simulink library "LIB_Quad_Com"  (Simulink 7.6)
settings: Solver=ode45  StartTime=0.0  StopTime=10.0  RelTol=1e-3
libraries: simulink x5
settings Model: Creator=Thomas  LastModifiedBy=Administrator

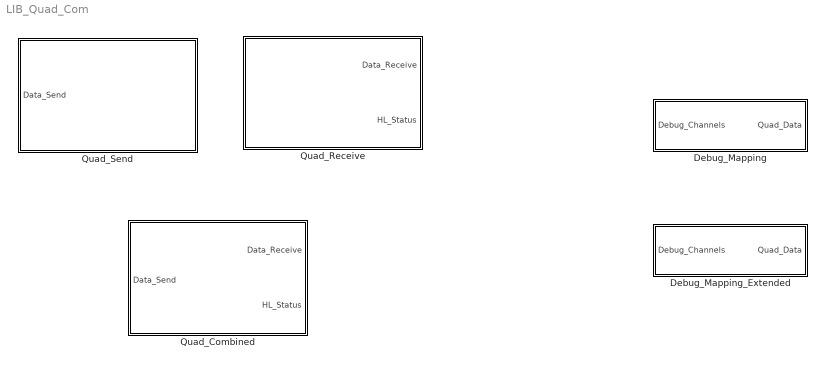
== system LIB_Quad_Com ==
  Debug_Mapping : Subsystem
  Debug_Mapping_Extended : Subsystem
  Quad_Combined : Subsystem  mask{baudrate=250000}
      mask Display:
      | image(imread('hummingbird.jpg'),[.15, .15, .7, .7],'on'),
      | port_label('input',1,'u'),
      | port_label('output',1,'y'),
      | port_label('output',2,'Status')
  Quad_Receive : Subsystem  mask{baudrate=250000}
      mask Display:
      | image(imread('hummingbird.jpg'),[.15, .15, .7, .7],'on'),
      | port_label('output',1,'y'),
      | port_label('output',2,'Status')
  Quad_Send : Subsystem  mask{baudrate=250000}
      mask Display:
      | image(imread('hummingbird.jpg'),[.15, .15, .7, .7],'on'),
      | port_label('input',1,'u')

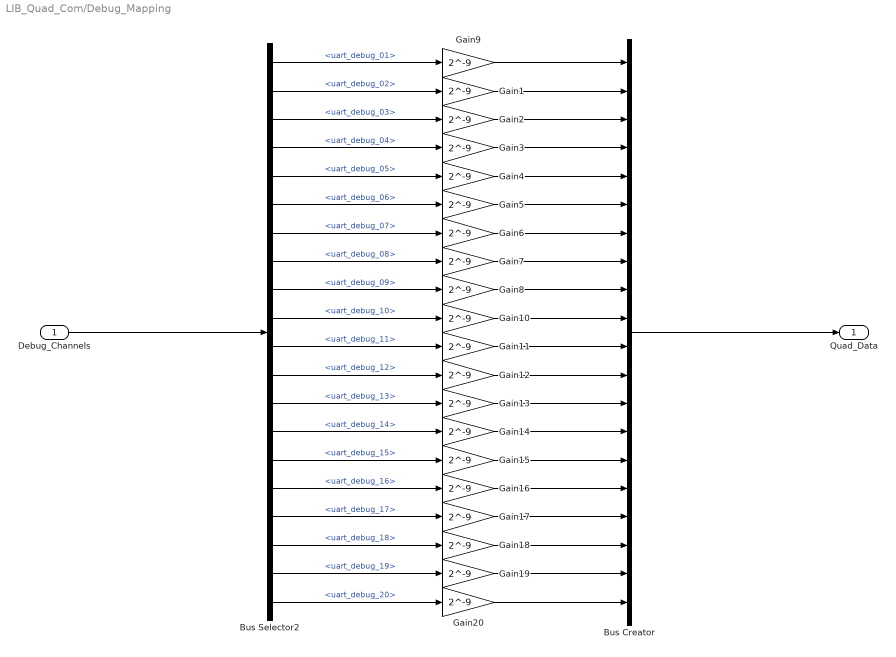
== system LIB_Quad_Com/Debug_Mapping ==
  Debug_Channels : Inport
  Bus Creator : BusCreator  Inputs=20
  Bus Selector2 : BusSelector  OutputSignals=uart_debug_01,uart_debug_02,uart_debug_03,uart_debug_04,uart_debug_05,uart_debug_06,uart_debug_07,uart_debug_08,uart_debug_09,uart_debug_10,uart_debug_11,uart_debug_12,uart_debug_13,uart_debug_14,uart_debug_15,uart_debug_16,uart_debug_17,uart_debug_18,uart_debug_19,uart_debug_20
  Gain{1..20} (20 alike) : Gain  Gain=2^-9  OutDataTypeStr=double
  Quad_Data : Outport
  wires:
  Gain20/1 -> Bus Creator/20
  Gain19/1 -> Bus Creator/19
  Gain18/1 -> Bus Creator/18
  Gain17/1 -> Bus Creator/17
  Gain16/1 -> Bus Creator/16
  Gain15/1 -> Bus Creator/15
  Gain14/1 -> Bus Creator/14
  Gain13/1 -> Bus Creator/13
  Gain12/1 -> Bus Creator/12
  Gain11/1 -> Bus Creator/11
  Gain10/1 -> Bus Creator/10
  Gain8/1 -> Bus Creator/9
  Gain7/1 -> Bus Creator/8
  Gain6/1 -> Bus Creator/7
  Gain5/1 -> Bus Creator/6
  Gain4/1 -> Bus Creator/5
  Gain3/1 -> Bus Creator/4
  Gain2/1 -> Bus Creator/3
  Gain1/1 -> Bus Creator/2
  Gain9/1 -> Bus Creator/1
  Bus Selector2/20 -> Gain20/1  "<uart_debug_20>"
  Bus Selector2/19 -> Gain19/1  "<uart_debug_19>"
  Bus Selector2/18 -> Gain18/1  "<uart_debug_18>"
  Bus Selector2/17 -> Gain17/1  "<uart_debug_17>"
  Bus Selector2/16 -> Gain16/1  "<uart_debug_16>"
  Bus Selector2/15 -> Gain15/1  "<uart_debug_15>"
  Bus Selector2/14 -> Gain14/1  "<uart_debug_14>"
  Bus Selector2/13 -> Gain13/1  "<uart_debug_13>"
  Bus Selector2/12 -> Gain12/1  "<uart_debug_12>"
  Bus Selector2/11 -> Gain11/1  "<uart_debug_11>"
  Bus Selector2/10 -> Gain10/1  "<uart_debug_10>"
  Bus Selector2/9 -> Gain8/1  "<uart_debug_09>"
  Bus Selector2/8 -> Gain7/1  "<uart_debug_08>"
  Bus Selector2/7 -> Gain6/1  "<uart_debug_07>"
  Bus Selector2/6 -> Gain5/1  "<uart_debug_06>"
  Bus Selector2/5 -> Gain4/1  "<uart_debug_05>"
  Bus Selector2/4 -> Gain3/1  "<uart_debug_04>"
  Bus Selector2/3 -> Gain2/1  "<uart_debug_03>"
  Bus Selector2/2 -> Gain1/1  "<uart_debug_02>"
  Bus Selector2/1 -> Gain9/1  "<uart_debug_01>"
  Debug_Channels/1 -> Bus Selector2/1
  Bus Creator/1 -> Quad_Data/1

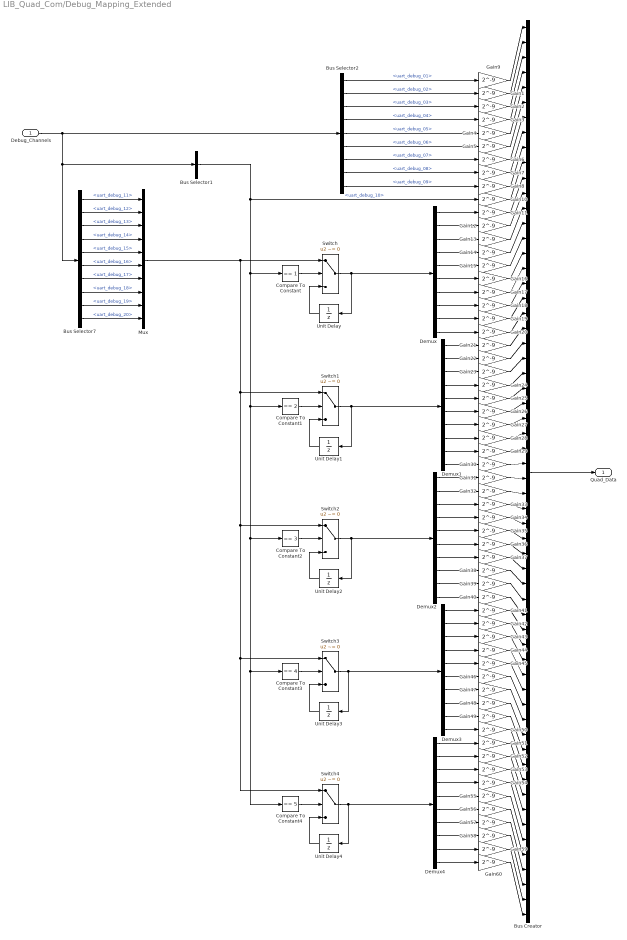
== system LIB_Quad_Com/Debug_Mapping_Extended ==
  Debug_Channels : Inport
  Bus Creator : BusCreator  Inputs=60
  Bus Selector1 : BusSelector  OutputSignals=uart_debug_10
  Bus Selector2 : BusSelector  OutputSignals=uart_debug_01,uart_debug_02,uart_debug_03,uart_debug_04,uart_debug_05,uart_debug_06,uart_debug_07,uart_debug_08,uart_debug_09
  Bus Selector7 : BusSelector  OutputSignals=uart_debug_11,uart_debug_12,uart_debug_13,uart_debug_14,uart_debug_15,uart_debug_16,uart_debug_17,uart_debug_18,uart_debug_19,uart_debug_20
  Compare To Constant : simulink/Logic and Bit Operations/Compare To Constant  SystemSampleTime=-1  relop===  const=1  LogicOutDataTypeMode=uint8  ZeroCross=off
  Compare To Constant1 : simulink/Logic and Bit Operations/Compare To Constant  SystemSampleTime=-1  relop===  const=2  LogicOutDataTypeMode=uint8  ZeroCross=off
  Compare To Constant2 : simulink/Logic and Bit Operations/Compare To Constant  SystemSampleTime=-1  relop===  const=3  LogicOutDataTypeMode=uint8  ZeroCross=off
  Compare To Constant3 : simulink/Logic and Bit Operations/Compare To Constant  SystemSampleTime=-1  relop===  const=4  LogicOutDataTypeMode=uint8  ZeroCross=off
  Compare To Constant4 : simulink/Logic and Bit Operations/Compare To Constant  SystemSampleTime=-1  relop===  const=5  LogicOutDataTypeMode=uint8  ZeroCross=off
  Demux{,1..4} (5 alike) : Demux  Outputs=10
  Gain{1..60} (60 alike) : Gain  Gain=2^-9  OutDataTypeStr=double
  Mux : Mux  Inputs=10
  Switch{,1..4} (5 alike) : Switch  Criteria=u2 ~= 0
  Unit Delay{,1..4} (5 alike) : UnitDelay  SampleTime=-1
  Quad_Data : Outport
  wires:
  Gain9/1 -> Bus Creator/1
  Bus Creator/1 -> Quad_Data/1
  Unit Delay4/1 -> Switch4/3
  Switch4/1 -> Demux4/1, Unit Delay4/1
  Compare To Constant4/1 -> Switch4/2
  Unit Delay3/1 -> Switch3/3
  Switch3/1 -> Demux3/1, Unit Delay3/1
  Compare To Constant3/1 -> Switch3/2
  Unit Delay2/1 -> Switch2/3
  Switch2/1 -> Demux2/1, Unit Delay2/1
  Compare To Constant2/1 -> Switch2/2
  Unit Delay1/1 -> Switch1/3
  Switch1/1 -> Demux1/1, Unit Delay1/1
  Compare To Constant1/1 -> Switch1/2
  Unit Delay/1 -> Switch/3
  Switch/1 -> Unit Delay/1, Demux/1
  Compare To Constant/1 -> Switch/2
  Demux4/10 -> Gain60/1
  Demux4/9 -> Gain59/1
  Demux4/8 -> Gain58/1
  Demux4/7 -> Gain57/1
  Demux4/6 -> Gain56/1
  Demux4/5 -> Gain55/1
  Demux4/4 -> Gain54/1
  Demux4/3 -> Gain53/1
  Demux4/2 -> Gain52/1
  Demux4/1 -> Gain51/1
  Demux3/10 -> Gain50/1
  Demux3/9 -> Gain49/1
  Demux3/8 -> Gain48/1
  Demux3/7 -> Gain47/1
  Demux3/6 -> Gain46/1
  Demux3/5 -> Gain45/1
  Demux3/4 -> Gain44/1
  Demux3/3 -> Gain43/1
  Demux3/2 -> Gain42/1
  Demux3/1 -> Gain41/1
  Demux2/10 -> Gain40/1
  Demux2/9 -> Gain39/1
  Demux2/8 -> Gain38/1
  Demux2/7 -> Gain37/1
  Demux2/6 -> Gain36/1
  Demux2/5 -> Gain35/1
  Demux2/4 -> Gain34/1
  Demux2/3 -> Gain33/1
  Demux2/2 -> Gain32/1
  Demux2/1 -> Gain31/1
  Demux1/10 -> Gain30/1
  Demux1/9 -> Gain29/1
  Demux1/8 -> Gain28/1
  Demux1/7 -> Gain27/1
  Demux1/6 -> Gain26/1
  Demux1/5 -> Gain25/1
  Demux1/4 -> Gain24/1
  Demux1/3 -> Gain23/1
  Demux1/2 -> Gain22/1
  Demux1/1 -> Gain21/1
  Demux/10 -> Gain20/1
  Demux/9 -> Gain19/1
  Demux/8 -> Gain18/1
  Demux/7 -> Gain17/1
  Demux/6 -> Gain16/1
  Demux/5 -> Gain15/1
  Demux/4 -> Gain14/1
  Demux/3 -> Gain13/1
  Demux/2 -> Gain12/1
  Demux/1 -> Gain11/1
  Bus Selector2/9 -> Gain8/1  "<uart_debug_09>"
  Bus Selector2/8 -> Gain7/1  "<uart_debug_08>"
  Bus Selector2/7 -> Gain6/1  "<uart_debug_07>"
  Bus Selector2/6 -> Gain5/1  "<uart_debug_06>"
  Bus Selector2/5 -> Gain4/1  "<uart_debug_05>"
  Bus Selector2/4 -> Gain3/1  "<uart_debug_04>"
  Bus Selector2/3 -> Gain2/1  "<uart_debug_03>"
  Bus Selector2/2 -> Gain1/1  "<uart_debug_02>"
  Bus Selector2/1 -> Gain9/1  "<uart_debug_01>"
  Bus Selector1/1 -> Compare To Constant4/1, Compare To Constant3/1, Compare To Constant2/1, Compare To Constant1/1, Compare To Constant/1, Gain10/1  "<uart_debug_10>"
  Mux/1 -> Switch4/1, Switch3/1, Switch2/1, Switch1/1, Switch/1
  Bus Selector7/10 -> Mux/10  "<uart_debug_20>"
  Bus Selector7/9 -> Mux/9  "<uart_debug_19>"
  Bus Selector7/8 -> Mux/8  "<uart_debug_18>"
  Bus Selector7/7 -> Mux/7  "<uart_debug_17>"
  Bus Selector7/6 -> Mux/6  "<uart_debug_16>"
  Bus Selector7/5 -> Mux/5  "<uart_debug_15>"
  Bus Selector7/4 -> Mux/4  "<uart_debug_14>"
  Bus Selector7/3 -> Mux/3  "<uart_debug_13>"
  Bus Selector7/2 -> Mux/2  "<uart_debug_12>"
  Bus Selector7/1 -> Mux/1  "<uart_debug_11>"
  Debug_Channels/1 -> Bus Selector1/1, Bus Selector7/1, Bus Selector2/1
  Gain1/1 -> Bus Creator/2
  Gain2/1 -> Bus Creator/3
  Gain3/1 -> Bus Creator/4
  Gain4/1 -> Bus Creator/5
  Gain5/1 -> Bus Creator/6
  Gain6/1 -> Bus Creator/7
  Gain7/1 -> Bus Creator/8
  Gain8/1 -> Bus Creator/9
  Gain10/1 -> Bus Creator/10
  Gain11/1 -> Bus Creator/11
  Gain12/1 -> Bus Creator/12
  Gain13/1 -> Bus Creator/13
  Gain14/1 -> Bus Creator/14
  Gain15/1 -> Bus Creator/15
  Gain16/1 -> Bus Creator/16
  Gain17/1 -> Bus Creator/17
  Gain18/1 -> Bus Creator/18
  Gain19/1 -> Bus Creator/19
  Gain20/1 -> Bus Creator/20
  Gain21/1 -> Bus Creator/21
  Gain22/1 -> Bus Creator/22
  Gain23/1 -> Bus Creator/23
  Gain24/1 -> Bus Creator/24
  Gain25/1 -> Bus Creator/25
  Gain26/1 -> Bus Creator/26
  Gain27/1 -> Bus Creator/27
  Gain28/1 -> Bus Creator/28
  Gain29/1 -> Bus Creator/29
  Gain30/1 -> Bus Creator/30
  Gain31/1 -> Bus Creator/31
  Gain32/1 -> Bus Creator/32
  Gain33/1 -> Bus Creator/33
  Gain34/1 -> Bus Creator/34
  Gain35/1 -> Bus Creator/35
  Gain36/1 -> Bus Creator/36
  Gain37/1 -> Bus Creator/37
  Gain38/1 -> Bus Creator/38
  Gain39/1 -> Bus Creator/39
  Gain40/1 -> Bus Creator/40
  Gain41/1 -> Bus Creator/41
  Gain42/1 -> Bus Creator/42
  Gain43/1 -> Bus Creator/43
  Gain44/1 -> Bus Creator/44
  Gain45/1 -> Bus Creator/45
  Gain46/1 -> Bus Creator/46
  Gain47/1 -> Bus Creator/47
  Gain48/1 -> Bus Creator/48
  Gain49/1 -> Bus Creator/49
  Gain50/1 -> Bus Creator/50
  Gain51/1 -> Bus Creator/51
  Gain52/1 -> Bus Creator/52
  Gain53/1 -> Bus Creator/53
  Gain54/1 -> Bus Creator/54
  Gain55/1 -> Bus Creator/55
  Gain56/1 -> Bus Creator/56
  Gain57/1 -> Bus Creator/57
  Gain58/1 -> Bus Creator/58
  Gain59/1 -> Bus Creator/59
  Gain60/1 -> Bus Creator/60

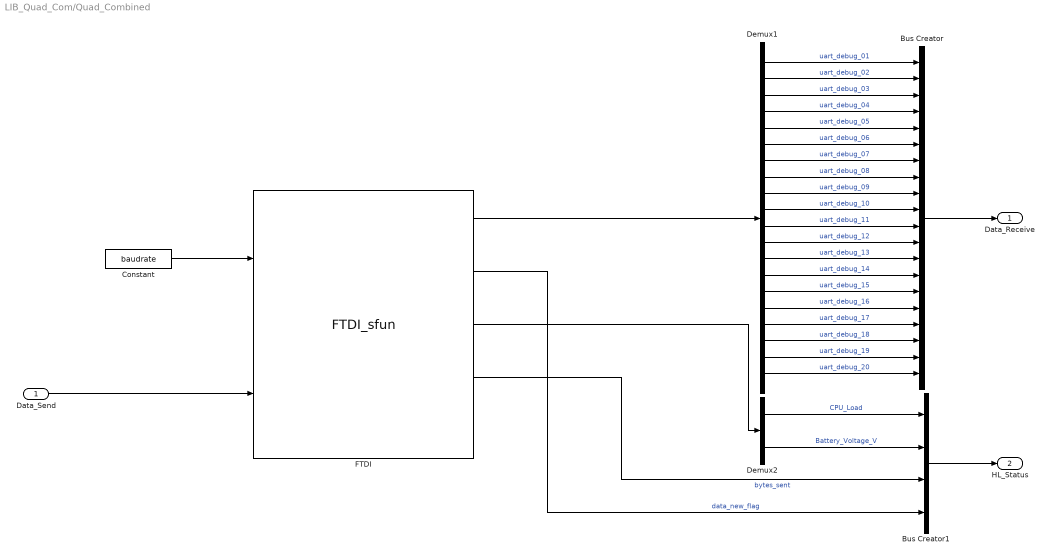
== system LIB_Quad_Com/Quad_Combined ==
  Data_Send : Inport  PortDimensions=[12 1]
  Bus Creator : BusCreator  Inputs=20
  Bus Creator1 : BusCreator
  Constant : Constant  Value=baudrate  OutDataTypeStr=int32  SampleTime=0.02
  Demux1 : Demux  Outputs=20
  Demux2 : Demux  Outputs=2
  FTDI : S-Function  InitFcn=try, set_param(gcb,'FunctionName','FTDI_sfun'), end  FunctionName=FTDI_sfun  SFunctionModules=FTDI_receive_sfun_wrapper ftditools  WizardData=DataTag0  EnableBusSupport=off  mask(S-Function Builder){}
      mask help: The S-Function Builder block creates a wrapper C-MEX S-function from your supplied C code with multiple input ports, output ports, and a variable number of scalar, vector, or matrix parameters. The input and output ports can propagate Simulink built-in data types, fixed-point datatypes, complex, frame, 1-D, and 2-D signals. This block also supports discrete and continuous states of type real. You can optionally have the block generate a TLC file to be used with Real-Time Workshop for code generation.
      mask init:
      | val = [[.9  0.75 0.75 1 1 .9 .9 1]',[1 1 0.75 0.75 .9 .9 1 .9]'];try , sys = get_param(gcb,'SfunBuilderFcnName');if isempty(sys), sys = get_param(gcb,'FunctionName'); end,catch, sys = get_param(gcb,'FunctionName'); end
      settings: CopyFcn=set_param(gcbh,'LinkStatus','none')  PreSaveFcn=try, set_param(gcb,'FunctionName','FTDI_sfun'), end  OpenFcn=sfunctionwizard(gcbh)
      mask Display: plot(val(:,1),val(:,2)),disp(sys), port_label('input',1,'set_BaudRate'), port_label('input',2,'data_send'), port_label('output',1,'data_out'), port_label('output',2,'data_new_flag'), port_label('output',3,'HL_Status'), port_label('output',4,'bytes_sent')
  Data_Receive : Outport
  HL_Status : Outport  Port=2
  wires:
  Data_Send/1 -> FTDI/2
  Constant/1 -> FTDI/1
  FTDI/2 -> Bus Creator1/4  "data_new_flag"
  FTDI/1 -> Demux1/1
  Demux1/1 -> Bus Creator/1  "uart_debug_01"
  Demux1/3 -> Bus Creator/3  "uart_debug_03"
  Demux1/2 -> Bus Creator/2  "uart_debug_02"
  Demux1/4 -> Bus Creator/4  "uart_debug_04"
  Demux1/5 -> Bus Creator/5  "uart_debug_05"
  Demux1/6 -> Bus Creator/6  "uart_debug_06"
  Demux1/7 -> Bus Creator/7  "uart_debug_07"
  Demux1/8 -> Bus Creator/8  "uart_debug_08"
  Demux1/9 -> Bus Creator/9  "uart_debug_09"
  Demux1/10 -> Bus Creator/10  "uart_debug_10"
  Demux1/11 -> Bus Creator/11  "uart_debug_11"
  Demux1/12 -> Bus Creator/12  "uart_debug_12"
  Demux1/13 -> Bus Creator/13  "uart_debug_13"
  Demux1/14 -> Bus Creator/14  "uart_debug_14"
  Demux1/15 -> Bus Creator/15  "uart_debug_15"
  Demux1/16 -> Bus Creator/16  "uart_debug_16"
  Demux1/17 -> Bus Creator/17  "uart_debug_17"
  Demux1/18 -> Bus Creator/18  "uart_debug_18"
  Demux1/19 -> Bus Creator/19  "uart_debug_19"
  Demux1/20 -> Bus Creator/20  "uart_debug_20"
  Bus Creator/1 -> Data_Receive/1
  Demux2/1 -> Bus Creator1/1  "CPU_Load"
  Demux2/2 -> Bus Creator1/2  "Battery_Voltage_V"
  Bus Creator1/1 -> HL_Status/1
  FTDI/4 -> Bus Creator1/3  "bytes_sent"
  FTDI/3 -> Demux2/1

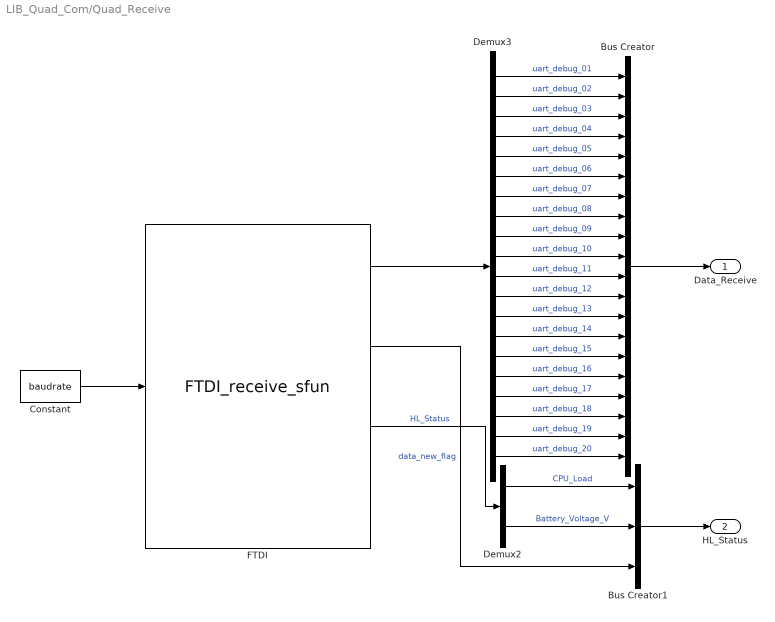
== system LIB_Quad_Com/Quad_Receive ==
  Bus Creator : BusCreator  Inputs=20
  Bus Creator1 : BusCreator  Inputs=3
  Constant : Constant  Value=baudrate  OutDataTypeStr=int32  SampleTime=0.02
  Demux2 : Demux  Outputs=2
  Demux3 : Demux  Outputs=20
  FTDI : S-Function  InitFcn=try, set_param(gcb,'FunctionName','FTDI_receive_sfun'), end  FunctionName=FTDI_receive_sfun  SFunctionModules=FTDI_receive_sfun_wrapper ftditools  WizardData=DataTag1  EnableBusSupport=off  mask(S-Function Builder){}
      mask help: The S-Function Builder block creates a wrapper C-MEX S-function from your supplied C code with multiple input ports, output ports, and a variable number of scalar, vector, or matrix parameters. The input and output ports can propagate Simulink built-in data types, fixed-point datatypes, complex, frame, 1-D, and 2-D signals. This block also supports discrete and continuous states of type real. You can optionally have the block generate a TLC file to be used with Real-Time Workshop for code generation.
      mask init: same as LIB_Quad_Com/Quad_Combined/FTDI
      settings: CopyFcn=set_param(gcbh,'LinkStatus','none')  PreSaveFcn=try, set_param(gcb,'FunctionName','FTDI_receive_sfun'), end  OpenFcn=sfunctionwizard(gcbh)
      mask Display: plot(val(:,1),val(:,2)),disp(sys), port_label('input',1,'BaudRate'), port_label('output',1,'data_out'), port_label('output',2,'data_new_flag'), port_label('output',3,'HL_Status')
  Data_Receive : Outport
  HL_Status : Outport  Port=2
  wires:
  Demux2/1 -> Bus Creator1/1  "CPU_Load"
  Demux2/2 -> Bus Creator1/2  "Battery_Voltage_V"
  Bus Creator1/1 -> HL_Status/1
  Bus Creator/1 -> Data_Receive/1
  Demux3/20 -> Bus Creator/20  "uart_debug_20"
  Demux3/19 -> Bus Creator/19  "uart_debug_19"
  Demux3/18 -> Bus Creator/18  "uart_debug_18"
  Demux3/17 -> Bus Creator/17  "uart_debug_17"
  Demux3/16 -> Bus Creator/16  "uart_debug_16"
  Demux3/15 -> Bus Creator/15  "uart_debug_15"
  Demux3/14 -> Bus Creator/14  "uart_debug_14"
  Demux3/13 -> Bus Creator/13  "uart_debug_13"
  Demux3/12 -> Bus Creator/12  "uart_debug_12"
  Demux3/11 -> Bus Creator/11  "uart_debug_11"
  Demux3/10 -> Bus Creator/10  "uart_debug_10"
  Demux3/9 -> Bus Creator/9  "uart_debug_09"
  Demux3/8 -> Bus Creator/8  "uart_debug_08"
  Demux3/7 -> Bus Creator/7  "uart_debug_07"
  Demux3/6 -> Bus Creator/6  "uart_debug_06"
  Demux3/5 -> Bus Creator/5  "uart_debug_05"
  Demux3/4 -> Bus Creator/4  "uart_debug_04"
  Demux3/2 -> Bus Creator/2  "uart_debug_02"
  Demux3/3 -> Bus Creator/3  "uart_debug_03"
  Demux3/1 -> Bus Creator/1  "uart_debug_01"
  FTDI/1 -> Demux3/1
  FTDI/2 -> Bus Creator1/3  "data_new_flag"
  Constant/1 -> FTDI/1
  FTDI/3 -> Demux2/1  "HL_Status"

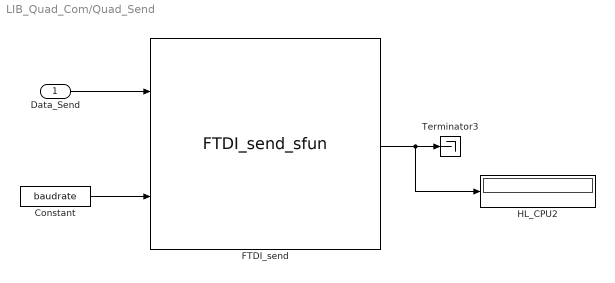
== system LIB_Quad_Com/Quad_Send ==
  Data_Send : Inport  PortDimensions=[12 1]
  Constant : Constant  Value=baudrate  OutDataTypeStr=int32
  FTDI_send : S-Function  InitFcn=try, set_param(gcb,'FunctionName','FTDI_send_sfun'), end  FunctionName=FTDI_send_sfun  SFunctionModules=FTDI_send_sfun_wrapper ftditools  WizardData=DataTag2  EnableBusSupport=off  mask(S-Function Builder){}
      mask help: The S-Function Builder block creates a wrapper C-MEX S-function from your supplied C code with multiple input ports, output ports, and a variable number of scalar, vector, or matrix parameters. The input and output ports can propagate Simulink built-in data types, fixed-point datatypes, complex, frame, 1-D, and 2-D signals. This block also supports discrete and continuous states of type real. You can optionally have the block generate a TLC file to be used with Real-Time Workshop for code generation.
      mask init: same as LIB_Quad_Com/Quad_Combined/FTDI
      settings: CopyFcn=set_param(gcbh,'LinkStatus','none')  PreSaveFcn=try, set_param(gcb,'FunctionName','FTDI_send_sfun'), end  OpenFcn=sfunctionwizard(gcbh)
      mask Display: plot(val(:,1),val(:,2)),disp(sys), port_label('input',1,'data_send'), port_label('input',2,'BaudRate'), port_label('output',1,'bytes_sent')
  HL_CPU2 : Display
  Terminator3 : Terminator
  wires:
  FTDI_send/1 -> HL_CPU2/1, Terminator3/1
  Constant/1 -> FTDI_send/2
  Data_Send/1 -> FTDI_send/1
